simulink model "Simulation"  (R2018a)
settings: Solver=VariableStepAuto  StartTime=0.0  StopTime=10  FixedStep=1e-6  MaxStep=Tsc  RelTol=1e-3  EnableMultiTasking=on
InitFcn:
  | clc
  | close all
  | clear all
  | 
  | %Vector-space-decomposition transform (2)
  | D = 2/6*[cos(0) cos(1*pi/3) cos(2*pi/3) cos(3*pi/3) cos(4*pi/3) cos(5*pi/3);
  |         sin(0) sin(1*pi/3) sin(2*pi/3) sin(3*pi/3) sin(4*pi/3) sin(5*pi/3);
  |         cos(2*0) cos(2*pi/3) cos(4*pi/3) cos(6*pi/3) cos(8*pi/3) cos(10*pi/3);
  |         sin(2*0) sin(2*pi/3) sin(4*pi/3) sin(6*pi/3) sin(8*pi/3) sin(10*pi/3);
  |         1/2 1/2  1/2 1/2 1/2 1/2;
  |         1/2 -1/2 1/2 -1/2 1/2 -1/2];
  | 
  | %Control sampling period
  | Tsc = 1e-4;
  | 
  | %Parameters of six-phase induction machine (other than stator resistance):
  | P=2; %Number of machine pole pairs
  | Lm=284e-3; %alpha-beta magnetizing inductance (mH)
  | Rr=2.9; %alpha-beta rotor resistance (ohm)
  | Lls=10e-3; %alpha-beta stator leakage inductance (mH)
  | Llr=21e-3; %alpha-beta rotor leakage inductance (mH)
  | Lxy=4.52e-3; %xy stator inductance (mH)
  | L0=24.5e-3; %0- stator inductance (mH)
  | J=0.0261; %Inertia (Kg*m^2)
  | f=0.0033; %Friction coefficient (N*m*s)
  | Ls = Lls+Lm; Lr = Llr+Lm;  %alpha-beta self-inductances (mH)
undefined symbols (not defined in the file): DiscIntNeverNeededParam
libraries: powerlib x37, simulink x20, simulink_extras x7
(part 3 of 3)

== system Simulation/Motor Control and Resistance Estimation/Proposed method/Generation of time sequence for injection/Time delay 3/Detect rising edge ==
  In : Inport
  Compare To Constant : simulink/Logic and Bit Operations/Compare To Constant  relop=>=  const=1  OutDataTypeStr=boolean
  Compare To Constant1 : simulink/Logic and Bit Operations/Compare To Constant  relop=<  const=1  OutDataTypeStr=boolean
  Logical Operator : Logic  AllPortsSameDT=off  OutDataTypeStr=boolean
  delay : UnitDelay  SampleTime=-1
  Out : Outport
  wires:
  delay/1 -> Compare To Constant1/1
  Logical Operator/1 -> Out/1
  In/1 -> Compare To Constant/1, delay/1
  Compare To Constant/1 -> Logical Operator/1
  Compare To Constant1/1 -> Logical Operator/2

== system Simulation/Motor Control and Resistance Estimation/Proposed method/R estimation/Equations (10) & (11)/Va ==
  V : Inport
  S&H 0 : Subsystem
  S&H 2 : Subsystem
  Sum1 : Sum  Inputs=+-  SaturateOnIntegerOverflow=on
  DVa_2 : Outport
  wires:
  V/1 -> S&H 2/1(In), S&H 0/1(In)
  S&H 2/1(Out) -> Sum1/1
  Sum1/1 -> DVa_2/1
  S&H 0/1(Out) -> Sum1/2
  [Instant0] -> S&H 0/2(trigger)
  [Instant2] -> S&H 2/2(trigger)

== system Simulation/Motor Control and Resistance Estimation/Proposed method/R estimation/Equations (10) & (11)/Vb ==
  V : Inport
  S&H 0 : Subsystem
  S&H 1 : Subsystem
  Sum1 : Sum  Inputs=+-  SaturateOnIntegerOverflow=on
  DVb_1 : Outport
  wires:
  [Instant1] -> S&H 1/2(trigger)
  [Instant0] -> S&H 0/2(trigger)
  S&H 0/1(Out) -> Sum1/2
  Sum1/1 -> DVb_1/1
  S&H 1/1(Out) -> Sum1/1
  V/1 -> S&H 0/1(In), S&H 1/1(In)

== system Simulation/Motor Control and Resistance Estimation/Proposed method/R estimation/Equations (10) & (11)/Vc ==
  V : Inport
  S&H 0 : Subsystem
  S&H 1 : Subsystem
  S&H 2 : Subsystem
  Sum1 : Sum  Inputs=+-  SaturateOnIntegerOverflow=on
  Sum2 : Sum  Inputs=+-  SaturateOnIntegerOverflow=on
  DVc_2 : Outport
  DVc_1 : Outport  Port=2
  wires:
  V/1 -> S&H 1/1(In), S&H 2/1(In), S&H 0/1(In)
  S&H 2/1(Out) -> Sum1/1
  Sum1/1 -> DVc_2/1
  S&H 0/1(Out) -> Sum2/2, Sum1/2
  [Instant0] -> S&H 0/2(trigger)
  [Instant2] -> S&H 2/2(trigger)
  Sum2/1 -> DVc_1/1
  S&H 1/1(Out) -> Sum2/1
  [Instant1] -> S&H 1/2(trigger)

== system Simulation/Motor Control and Resistance Estimation/Proposed method/R estimation/Equations (10) & (11)/Vd ==
  V : Inport
  S&H 0 : Subsystem
  S&H 1 : Subsystem
  S&H 2 : Subsystem
  Sum1 : Sum  Inputs=+-  SaturateOnIntegerOverflow=on
  Sum2 : Sum  Inputs=+-  SaturateOnIntegerOverflow=on
  DVd_2 : Outport
  DVd_1 : Outport  Port=2
  wires:
  [Instant2] -> S&H 2/2(trigger)
  [Instant0] -> S&H 0/2(trigger)
  S&H 0/1(Out) -> Sum2/2, Sum1/2
  Sum1/1 -> DVd_2/1
  S&H 2/1(Out) -> Sum1/1
  V/1 -> S&H 0/1(In), S&H 1/1(V), S&H 2/1(In)
  Sum2/1 -> DVd_1/1
  [Instant1] -> S&H 1/2(trigger)
  S&H 1/1(Out) -> Sum2/1

== system Simulation/Motor Control and Resistance Estimation/Proposed method/R estimation/Equations (10) & (11)/Ve ==
  V : Inport
  S&H 0 : Subsystem
  S&H 1 : Subsystem
  S&H 2 : Subsystem
  Sum1 : Sum  Inputs=+-  SaturateOnIntegerOverflow=on
  Sum2 : Sum  Inputs=+-  SaturateOnIntegerOverflow=on
  DVe_1 : Outport
  DVe_2 : Outport  Port=2
  wires:
  V/1 -> S&H 2/1(In), S&H 1/1(In), S&H 0/1(In)
  S&H 1/1(Out) -> Sum1/1
  Sum1/1 -> DVe_1/1
  S&H 0/1(Out) -> Sum2/2, Sum1/2
  [Instant0] -> S&H 0/2(trigger)
  [Instant1] -> S&H 1/2(trigger)
  [Instant2] -> S&H 2/2(trigger)
  S&H 2/1(Out) -> Sum2/1
  Sum2/1 -> DVe_2/1

== system Simulation/Motor Control and Resistance Estimation/Proposed method/R estimation/Equations (10) & (11)/Vf ==
  V : Inport
  S&H 0 : Subsystem
  S&H 1 : Subsystem
  S&H 2 : Subsystem
  Sum1 : Sum  Inputs=+-  SaturateOnIntegerOverflow=on
  Sum2 : Sum  Inputs=+-  SaturateOnIntegerOverflow=on
  DVf_1 : Outport
  DVf_2 : Outport  Port=2
  wires:
  Sum2/1 -> DVf_2/1
  S&H 2/1(Out) -> Sum2/1
  [Instant2] -> S&H 2/2(trigger)
  [Instant1] -> S&H 1/2(trigger)
  [Instant0] -> S&H 0/2(trigger)
  S&H 0/1(Out) -> Sum1/2, Sum2/2
  Sum1/1 -> DVf_1/1
  S&H 1/1(Out) -> Sum1/1
  V/1 -> S&H 0/1(In), S&H 1/1(In), S&H 2/1(In)

== system Simulation/Motor Control and Resistance Estimation/Speed control loop/Subsystem2/Estimation of rotor-flux position and speed/slip estimator ==
  Iqs : Inport
  Ids : Inport  Port=2
  Divide : Product  Inputs=*/
  Gain : Gain  Gain=Rr/Lr
  slip speed : Outport  VectorParamsAs1DForOutWhenUnconnected=off
  wires:
  Divide/1 -> slip speed/1
  Iqs/1 -> Gain/1
  Ids/1 -> Divide/2
  Gain/1 -> Divide/1

== system Simulation/Motor Control and Resistance Estimation/Speed control loop/Subsystem2/Inverse Park transformation/Inverse Park transform  ==
  dq : Inport
  sin_cos : Inport  Port=2
  Demux : Demux  Outputs=2
  Demux1 : Demux  Outputs=2
  Mux : Mux  Inputs=2
  Product{,1..3} (4 alike) : Product  InputSameDT=on  SaturateOnIntegerOverflow=on  OutDataTypeStr=Inherit: Same as first input
  Sum : Sum  Inputs=+-  InputSameDT=on  SaturateOnIntegerOverflow=on  OutDataTypeStr=Inherit: Same as first input
  Sum1 : Sum  InputSameDT=on  SaturateOnIntegerOverflow=on  OutDataTypeStr=Inherit: Same as first input
  ab : Outport  VectorParamsAs1DForOutWhenUnconnected=off
  wires:
  sin_cos/1 -> Demux1/1
  dq/1 -> Demux/1
  Sum1/1 -> Mux/2
  Demux1/1 -> Product1/1, Product3/1
  Demux1/2 -> Product2/1, Product/1
  Demux/2 -> Product1/2, Product2/2
  Demux/1 -> Product/2, Product3/2
  Mux/1 -> ab/1
  Sum/1 -> Mux/1
  Product1/1 -> Sum/2
  Product2/1 -> Sum1/2
  Product3/1 -> Sum1/1
  Product/1 -> Sum/1

== system Simulation/Motor Control and Resistance Estimation/Proposed method/R estimation/Equations (10) & (11)/Va/S&H 0 ==
  In : Inport
  trigger : Inport  Port=2
  Memory : UnitDelay  SampleTime=-1
  Switch : Switch  Threshold=0.5  SaturateOnIntegerOverflow=on
  Out : Outport
  wires:
  In/1 -> Switch/1
  Memory/1 -> Switch/3, Out/1
  Switch/1 -> Memory/1
  trigger/1 -> Switch/2

== system Simulation/Motor Control and Resistance Estimation/Proposed method/R estimation/Equations (10) & (11)/Va/S&H 2 ==
  In : Inport
  trigger : Inport  Port=2
  Memory : UnitDelay  SampleTime=-1
  Switch : Switch  Threshold=0.5  SaturateOnIntegerOverflow=on
  Out : Outport
  wires:
  trigger/1 -> Switch/2
  In/1 -> Switch/1
  Memory/1 -> Switch/3, Out/1
  Switch/1 -> Memory/1

== system Simulation/Motor Control and Resistance Estimation/Proposed method/R estimation/Equations (10) & (11)/Vb/S&H 0 ==
  In : Inport
  trigger : Inport  Port=2
  Memory : UnitDelay  SampleTime=-1
  Switch : Switch  Threshold=0.5  SaturateOnIntegerOverflow=on
  Out : Outport
  wires:
  trigger/1 -> Switch/2
  Switch/1 -> Memory/1
  Memory/1 -> Out/1, Switch/3
  In/1 -> Switch/1

== system Simulation/Motor Control and Resistance Estimation/Proposed method/R estimation/Equations (10) & (11)/Vb/S&H 1 ==
  In : Inport
  trigger : Inport  Port=2
  Memory : UnitDelay  SampleTime=-1
  Switch : Switch  Threshold=0.5  SaturateOnIntegerOverflow=on
  Out : Outport
  wires:
  Switch/1 -> Memory/1
  Memory/1 -> Out/1, Switch/3
  In/1 -> Switch/1
  trigger/1 -> Switch/2

== system Simulation/Motor Control and Resistance Estimation/Proposed method/R estimation/Equations (10) & (11)/Vc/S&H 0 ==
  In : Inport
  trigger : Inport  Port=2
  Memory : UnitDelay  SampleTime=-1
  Switch : Switch  Threshold=0.5  SaturateOnIntegerOverflow=on
  Out : Outport
  wires:
  In/1 -> Switch/1
  Memory/1 -> Switch/3, Out/1
  Switch/1 -> Memory/1
  trigger/1 -> Switch/2

== system Simulation/Motor Control and Resistance Estimation/Proposed method/R estimation/Equations (10) & (11)/Vc/S&H 1 ==
  In : Inport
  trigger : Inport  Port=2
  Memory : UnitDelay  SampleTime=-1
  Switch : Switch  Threshold=0.5  SaturateOnIntegerOverflow=on
  Out : Outport
  wires:
  Switch/1 -> Memory/1
  Memory/1 -> Out/1, Switch/3
  In/1 -> Switch/1
  trigger/1 -> Switch/2

== system Simulation/Motor Control and Resistance Estimation/Proposed method/R estimation/Equations (10) & (11)/Vc/S&H 2 ==
  In : Inport
  trigger : Inport  Port=2
  Memory : UnitDelay  SampleTime=-1
  Switch : Switch  Threshold=0.5  SaturateOnIntegerOverflow=on
  Out : Outport
  wires:
  trigger/1 -> Switch/2
  In/1 -> Switch/1
  Memory/1 -> Switch/3, Out/1
  Switch/1 -> Memory/1

== system Simulation/Motor Control and Resistance Estimation/Proposed method/R estimation/Equations (10) & (11)/Vd/S&H 0 ==
  In : Inport
  trigger : Inport  Port=2
  Memory : UnitDelay  SampleTime=-1
  Switch : Switch  Threshold=0.5  SaturateOnIntegerOverflow=on
  Out : Outport
  wires:
  trigger/1 -> Switch/2
  Switch/1 -> Memory/1
  Memory/1 -> Out/1, Switch/3
  In/1 -> Switch/1

== system Simulation/Motor Control and Resistance Estimation/Proposed method/R estimation/Equations (10) & (11)/Vd/S&H 1 ==
  V : Inport
  trigger : Inport  Port=2
  Memory : UnitDelay  SampleTime=-1
  Switch : Switch  Threshold=0.5  SaturateOnIntegerOverflow=on
  Out : Outport
  wires:
  Switch/1 -> Memory/1
  Memory/1 -> Out/1, Switch/3
  V/1 -> Switch/1
  trigger/1 -> Switch/2

== system Simulation/Motor Control and Resistance Estimation/Proposed method/R estimation/Equations (10) & (11)/Vd/S&H 2 ==
  In : Inport
  trigger : Inport  Port=2
  Memory : UnitDelay  SampleTime=-1
  Switch : Switch  Threshold=0.5  SaturateOnIntegerOverflow=on
  Out : Outport
  wires:
  Switch/1 -> Memory/1
  Memory/1 -> Out/1, Switch/3
  In/1 -> Switch/1
  trigger/1 -> Switch/2

== system Simulation/Motor Control and Resistance Estimation/Proposed method/R estimation/Equations (10) & (11)/Ve/S&H 0 ==
  In : Inport
  trigger : Inport  Port=2
  Memory : UnitDelay  SampleTime=-1
  Switch : Switch  Threshold=0.5  SaturateOnIntegerOverflow=on
  Out : Outport
  wires:
  In/1 -> Switch/1
  Memory/1 -> Switch/3, Out/1
  Switch/1 -> Memory/1
  trigger/1 -> Switch/2

== system Simulation/Motor Control and Resistance Estimation/Proposed method/R estimation/Equations (10) & (11)/Ve/S&H 1 ==
  In : Inport
  trigger : Inport  Port=2
  Memory : UnitDelay  SampleTime=-1
  Switch : Switch  Threshold=0.5  SaturateOnIntegerOverflow=on
  Out : Outport
  wires:
  trigger/1 -> Switch/2
  In/1 -> Switch/1
  Memory/1 -> Switch/3, Out/1
  Switch/1 -> Memory/1

== system Simulation/Motor Control and Resistance Estimation/Proposed method/R estimation/Equations (10) & (11)/Ve/S&H 2 ==
  In : Inport
  trigger : Inport  Port=2
  Memory : UnitDelay  SampleTime=-1
  Switch : Switch  Threshold=0.5  SaturateOnIntegerOverflow=on
  Out : Outport
  wires:
  trigger/1 -> Switch/2
  In/1 -> Switch/1
  Memory/1 -> Switch/3, Out/1
  Switch/1 -> Memory/1

== system Simulation/Motor Control and Resistance Estimation/Proposed method/R estimation/Equations (10) & (11)/Vf/S&H 0 ==
  In : Inport
  trigger : Inport  Port=2
  Memory : UnitDelay  SampleTime=-1
  Switch : Switch  Threshold=0.5  SaturateOnIntegerOverflow=on
  Out : Outport
  wires:
  trigger/1 -> Switch/2
  Switch/1 -> Memory/1
  Memory/1 -> Out/1, Switch/3
  In/1 -> Switch/1

== system Simulation/Motor Control and Resistance Estimation/Proposed method/R estimation/Equations (10) & (11)/Vf/S&H 1 ==
  In : Inport
  trigger : Inport  Port=2
  Memory : UnitDelay  SampleTime=-1
  Switch : Switch  Threshold=0.5  SaturateOnIntegerOverflow=on
  Out : Outport
  wires:
  Switch/1 -> Memory/1
  Memory/1 -> Out/1, Switch/3
  In/1 -> Switch/1
  trigger/1 -> Switch/2

== system Simulation/Motor Control and Resistance Estimation/Proposed method/R estimation/Equations (10) & (11)/Vf/S&H 2 ==
  In : Inport
  trigger : Inport  Port=2
  Memory : UnitDelay  SampleTime=-1
  Switch : Switch  Threshold=0.5  SaturateOnIntegerOverflow=on
  Out : Outport
  wires:
  Switch/1 -> Memory/1
  Memory/1 -> Out/1, Switch/3
  In/1 -> Switch/1
  trigger/1 -> Switch/2
